simulink model "dz_1_simul_model"  (R2026a)
settings: Solver=VariableStepAuto  StopTime=30
values from neighbouring files (symbols this model uses):
  g = 9.81    [dz_1_model.m]
  mass_quadrotor = 1.07    [dz_1_model.m]
undefined symbols (not defined in the file or in its folder): step_time
settings Model: Creator=vas77  LastModifiedBy=vas77
settings HardwareCC: ProdHWDeviceType=AMD->x86-64 (Windows64)
settings RTWCC: BuildConfiguration=Faster Runs

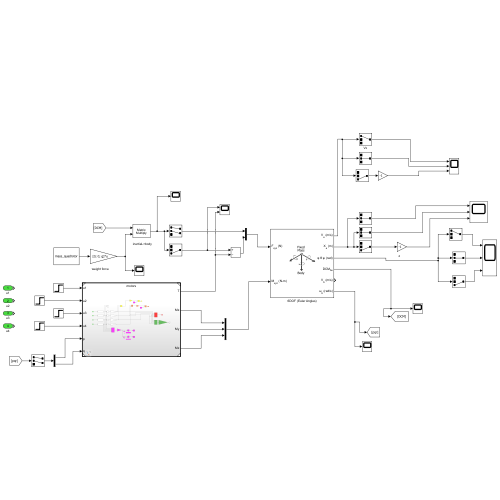
[thumbnail: Simulink's stored preview of the top-level diagram]
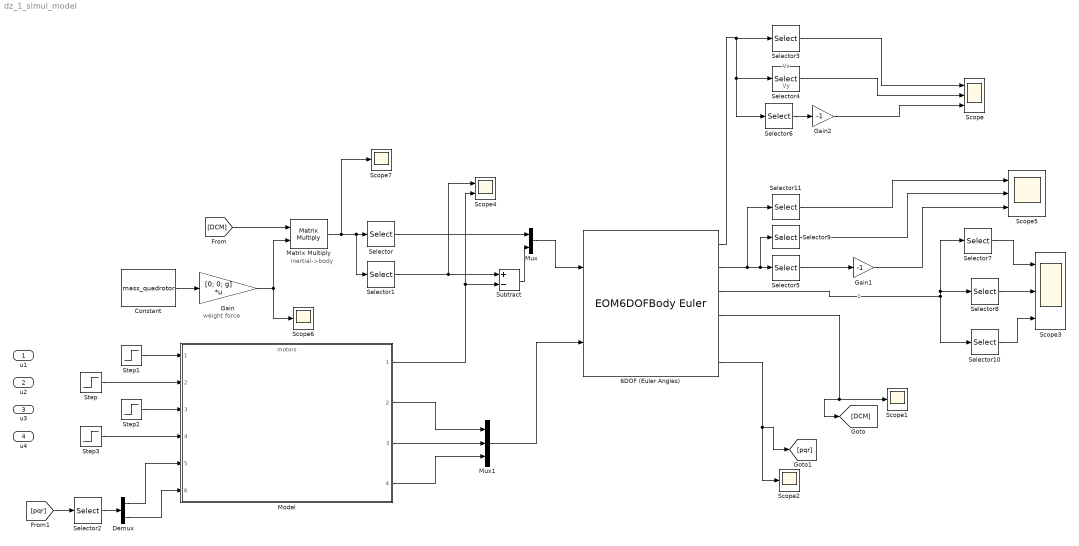
== system dz_1_simul_model ==
  note: Vx
  note: Vy
  note: z
  note: weight force
  note: inertial->body
  u1 : Inport
  u2 : Inport  Port=2
  u3 : Inport  Port=3
  u4 : Inport  Port=4
  6DOF (Euler Angles) : EOM6DOFBodyEuler  mass_0=mass_quadrotor
  Constant : Constant  Value=mass_quadrotor  VectorParams1D=off
  Demux : Demux  Outputs=2
  Gain : Gain  Gain=[0; 0; g]  Multiplication=Matrix(K*u)
  Gain1 : Gain  Gain=-1
  Gain2 : Gain  Gain=-1
  Matrix Multiply : Product  Multiplication=Matrix(*)
  Model : ModelReference  ModelNameDialog=motors.slx  SimulationMode=Normal  ModelReferenceVersion=1.12
  Mux : Mux  Inputs=2
  Mux1 : Mux  Inputs=3
  Scope : Scope  NumInputPorts=3
      settings: ActiveDisplayYMinimum=-13.567191607588207  ActiveDisplayYMaximum=122.10472444832429  YLabel=Altitude(m)
  Scope{1..2,6..7} (4 alike) : Scope
      Scope1 settings: ActiveDisplayYMinimum=-1.2499491050427127  ActiveDisplayYMaximum=1.2499943450047457
      Scope2 settings: ActiveDisplayYMinimum=-1  ActiveDisplayYMaximum=1  DataLoggingVariableName=ScopeData2
      Scope6 settings: ActiveDisplayYMinimum=5.1775949245841977  ActiveDisplayYMaximum=10.902189225640303  DataLoggingVariableName=ScopeData6
      Scope7 settings: ActiveDisplayYMinimum=-1  ActiveDisplayYMaximum=1  DataLoggingVariableName=ScopeData7
  Scope3 : Scope  NumInputPorts=3
      settings: ActiveDisplayYMinimum=-0.697882456363228  ActiveDisplayYMaximum=0.077542495151469756  DataLoggingVariableName=ScopeData3
  Scope4 : Scope  NumInputPorts=2
      settings: ActiveDisplayYMinimum=5.9584764482034869  ActiveDisplayYMaximum=15.675635410083268  DataLoggingVariableName=ScopeData4
  Scope5 : Scope  NumInputPorts=3
      settings: ActiveDisplayYMinimum=-13.145723051040948  ActiveDisplayYMaximum=118.31150745936758  YLabel=Altitude(m)  DataLoggingVariableName=ScopeData5
  Selector : Selector  IndexMode=Zero-based  InputPortWidth=3  IndexOptions=Index vector (dialog)  Indices=[0 1]  OutputSizes=1
  Selector{1,5..6,10} (4 alike) : Selector  IndexMode=Zero-based  InputPortWidth=3  IndexOptions=Index vector (dialog)  Indices=[2]  OutputSizes=1
  Selector{4,8..9,11} (4 alike) : Selector  IndexMode=Zero-based  InputPortWidth=3  IndexOptions=Index vector (dialog)  Indices=[1]  OutputSizes=1
  Selector2 : Selector  IndexMode=Zero-based  InputPortWidth=3  IndexOptions=Index vector (dialog)  Indices=[0 1]  OutputSizes=1
  Selector3 : Selector  IndexMode=Zero-based  InputPortWidth=3  IndexOptions=Index vector (dialog)  Indices=[0]  OutputSizes=1
  Selector7 : Selector  IndexMode=Zero-based  InputPortWidth=3  IndexOptions=Index vector (dialog)  Indices=[0]  OutputSizes=1
  Step : Step  Time=step_time  InitialValue=initial_val  FinalValue=final_val_u2  SampleTime=0
  Step1 : Step  Time=step_time  InitialValue=initial_val  FinalValue=final_val_u1  SampleTime=0
  Step2 : Step  Time=step_time  InitialValue=initial_val  FinalValue=final_val_u3  SampleTime=0
  Step3 : Step  Time=step_time  InitialValue=initial_val  FinalValue=final_val_u4  SampleTime=0
  Subtract : Sum  Inputs=+-
  wires:
  Constant/1 -> Gain/1
  [DCM] -> Matrix Multiply/1
  Gain/1 -> Matrix Multiply/2, Scope6/1
  Matrix Multiply/1 -> Scope7/1, Selector1/1, Selector/1
  Selector1/1 -> Scope4/1, Subtract/1
  Subtract/1 -> Mux/2
  Selector/1 -> Mux/1
  Model/1 -> Scope4/2, Subtract/2
  Mux/1 -> 6DOF (Euler Angles)/1
  Model/2 -> Mux1/1
  Model/3 -> Mux1/2
  Model/4 -> Mux1/3
  Mux1/1 -> 6DOF (Euler Angles)/2
  6DOF (Euler Angles)/4 -> [DCM], Scope1/1
  [pqr] -> Selector2/1
  Demux/1 -> Model/5
  Demux/2 -> Model/6
  Selector2/1 -> Demux/1
  6DOF (Euler Angles)/6 -> [pqr], Scope2/1
  6DOF (Euler Angles)/1 -> Selector6/1, Selector4/1, Selector3/1
  Selector5/1 -> Gain1/1
  6DOF (Euler Angles)/2 -> Selector11/1, Selector9/1, Selector5/1
  Selector6/1 -> Gain2/1
  Gain2/1 -> Scope/3
  Selector3/1 -> Scope/1
  Selector4/1 -> Scope/2
  Step1/1 -> Model/1
  Step2/1 -> Model/3
  6DOF (Euler Angles)/3 -> Selector7/1, Selector8/1, Selector10/1
  Selector7/1 -> Scope3/1
  Selector8/1 -> Scope3/2
  Selector10/1 -> Scope3/3
  Step3/1 -> Model/4
  Step/1 -> Model/2
  Selector11/1 -> Scope5/1
  Selector9/1 -> Scope5/2
  Gain1/1 -> Scope5/3
